simulink model "sampleModel1746"  (R2023a)
settings: Solver=VariableStepAuto  StartTime=0.0  StopTime=10.0  RelTol=1e-3
libraries: hdlsllib x2
settings Model: Creator=user1  LastModifiedBy=user1

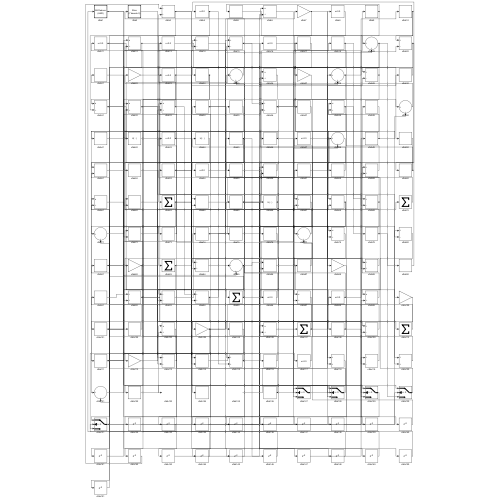
[thumbnail: Simulink's stored preview of the top-level diagram]
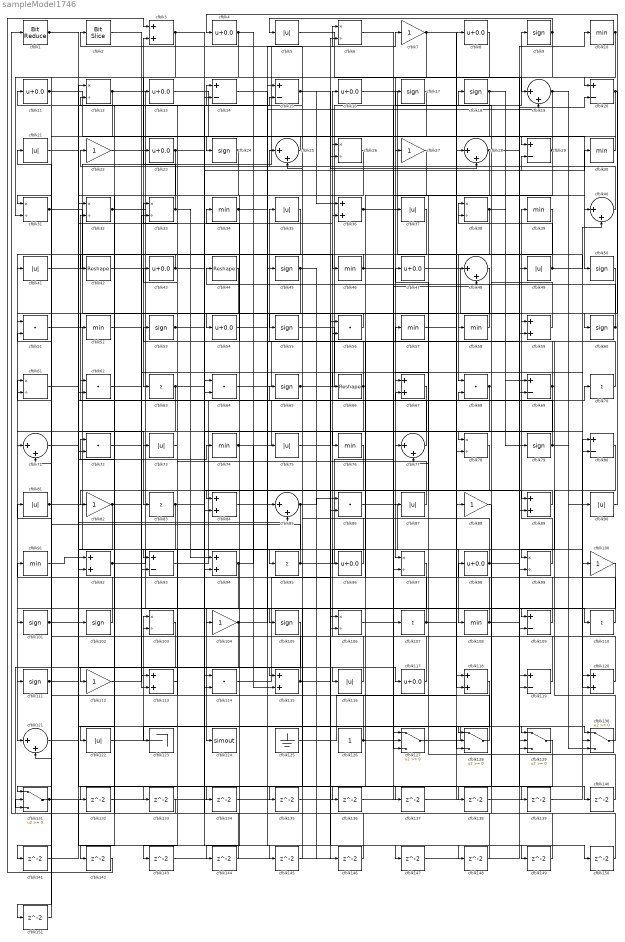
== system sampleModel1746 ==
  cfblk1 : hdlsllib/Logic and Bit Operations/Bit Reduce  mode=AND
  cfblk{10,30,34,39,46,52,57..58,74,76,91,108} (12 alike) : MinMax
  cfblk{7,22,27,82,88,100,104,112} (8 alike) : Gain
  cfblk{9,17..18,24,45,50,53,55,60,65,79,101..102,105,111} (15 alike) : Signum
  cfblk{6,12,26,31..33,38,61,78,97,99,103,106} (13 alike) : Product  Inputs=*/  RndMeth=Zero  SaturateOnIntegerOverflow=on
  cfblk{63,70,83,95,107,110} (6 alike) : Sum  Inputs=+
  cfblk{14..15,20,29,69,80,93,109,119} (9 alike) : Sum  Inputs=+-
  cfblk{4,8,11,13,16,23,43,47,54,96,98,117} (12 alike) : Bias  Bias=0.0  SaturateOnIntegerOverflow=off
  cfblk{3,36,59,67,84,89,92,94,113,115,118,120} (12 alike) : Sum
  cfblk{51,56,62,64,68,72,86,114} (8 alike) : DotProduct  OutDataTypeStr=Inherit: Inherit via internal rule
  cfblk{5,21,35,37,41,49,73,75,81,87,90,116,122} (13 alike) : Abs  SaturateOnIntegerOverflow=off
  cfblk{19,25,28,40,48,71,77,85,121} (9 alike) : Sum  Inputs=|++
  cfblk123 : Terminator
  cfblk124 : ToWorkspace  VariableName=simout  SaveFormat=Timeseries  SampleTime=-1
  cfblk125 : Ground
  cfblk126 : Constant  SampleTime=-1
  cfblk{127..131} (5 alike) : Switch  SaturateOnIntegerOverflow=off  InputSameDT=off
  cfblk{132..151} (20 alike) : Delay  SampleTime=1
  cfblk2 : hdlsllib/Logic and Bit Operations/Bit Slice  lidx=7  ridx=0
  cfblk42 : Reshape
  cfblk44 : Reshape
  cfblk66 : Reshape
  wires:
  cfblk8/1 -> cfblk97/1
  cfblk120/1 -> cfblk47/1
  cfblk24/1 -> cfblk52/1, cfblk132/1
  cfblk9/1 -> cfblk5/1, cfblk31/1
  cfblk69/1 -> cfblk35/1, cfblk86/2
  cfblk74/1 -> cfblk70/1, cfblk7/1
  cfblk99/1 -> cfblk39/1
  cfblk16/1 -> cfblk68/1
  cfblk32/1 -> cfblk109/1, cfblk64/2
  cfblk31/1 -> cfblk54/1, cfblk14/1
  cfblk91/1 -> cfblk92/1
  cfblk25/1 -> cfblk24/1
  cfblk40/1 -> cfblk22/1
  cfblk117/1 -> cfblk16/1
  cfblk104/1 -> cfblk57/1, cfblk110/1, cfblk133/1, cfblk134/1
  cfblk90/1 -> cfblk4/1
  cfblk65/1 -> cfblk9/1, cfblk97/2, cfblk128/3
  cfblk45/1 -> cfblk121/1, cfblk84/2, cfblk146/1
  cfblk125/1 -> cfblk28/1
  cfblk36/1 -> cfblk100/1, cfblk40/1
  cfblk60/1 -> cfblk44/1, cfblk51/1
  cfblk76/1 -> cfblk112/1
  cfblk12/1 -> cfblk66/1, cfblk62/2
  cfblk94/1 -> cfblk121/2, cfblk75/1
  cfblk107/1 -> cfblk8/1, cfblk72/1
  cfblk23/1 -> cfblk78/1, cfblk72/2
  cfblk35/1 -> cfblk111/1
  cfblk92/1 -> cfblk95/1, cfblk118/2
  cfblk4/1 -> cfblk63/1, cfblk115/2
  cfblk13/1 -> cfblk50/1
  cfblk28/1 -> cfblk67/1, cfblk20/2
  cfblk127/1 -> cfblk130/1
  cfblk58/1 -> cfblk26/1
  cfblk46/1 -> cfblk41/1, cfblk69/2
  cfblk39/1 -> cfblk77/1
  cfblk7/1 -> cfblk89/1, cfblk14/2
  cfblk33/1 -> cfblk3/2, cfblk94/1
  cfblk131/1 -> cfblk26/2, cfblk145/1
  cfblk53/1 -> cfblk109/2, cfblk149/1
  cfblk29/1 -> cfblk37/1, cfblk23/1
  cfblk81/1 -> cfblk120/1, cfblk93/1
  cfblk122/1 -> cfblk103/1
  cfblk15/1 -> cfblk28/2, cfblk36/1
  cfblk114/1 -> cfblk56/1
  cfblk59/1 -> cfblk17/1
  cfblk49/1 -> cfblk38/1, cfblk40/2
  cfblk41/1 -> cfblk6/1
  cfblk86/1 -> cfblk108/1
  cfblk38/1 -> cfblk58/1, cfblk69/1
  cfblk128/1 -> cfblk81/1
  cfblk62/1 -> cfblk113/1
  cfblk100/1 -> cfblk124/1
  cfblk17/1 -> cfblk71/1
  cfblk66/1 -> cfblk34/1, cfblk151/1
  cfblk55/1 -> cfblk107/1
  cfblk108/1 -> cfblk56/2, cfblk140/1
  cfblk19/1 -> cfblk29/1, cfblk90/1, cfblk94/2
  cfblk85/1 -> cfblk123/1, cfblk86/1, cfblk93/2
  cfblk105/1 -> cfblk131/1
  cfblk63/1 -> cfblk83/1, cfblk29/2, cfblk129/3
  cfblk68/1 -> cfblk78/2, cfblk96/1
  cfblk109/1 -> cfblk61/1
  cfblk57/1 -> cfblk30/1
  cfblk61/1 -> cfblk102/1
  cfblk30/1 -> cfblk27/1
  cfblk93/1 -> cfblk15/1
  cfblk82/1 -> cfblk92/2, cfblk116/1
  cfblk10/1 -> cfblk20/1, cfblk129/2
  cfblk56/1 -> cfblk55/1
  cfblk116/1 -> cfblk21/1
  cfblk44/1 -> cfblk122/1
  cfblk47/1 -> cfblk119/2
  cfblk77/1 -> cfblk32/2
  cfblk3/1 -> cfblk114/1, cfblk31/2, cfblk139/1
  cfblk51/1 -> cfblk114/2
  cfblk73/1 -> cfblk13/1
  cfblk101/1 -> cfblk67/2, cfblk129/1, cfblk36/2
  cfblk130/1 -> cfblk59/1
  cfblk14/1 -> cfblk85/1
  cfblk21/1 -> cfblk73/1
  cfblk121/1 -> cfblk85/2
  cfblk42/1 -> cfblk120/2
  cfblk72/1 -> cfblk68/2
  cfblk119/1 -> cfblk25/1
  cfblk113/1 -> cfblk53/1
  cfblk64/1 -> cfblk49/1
  cfblk27/1 -> cfblk76/1
  cfblk80/1 -> cfblk99/1
  cfblk115/1 -> cfblk62/1, cfblk150/1
  cfblk110/1 -> cfblk98/1
  cfblk83/1 -> cfblk113/2, cfblk15/2
  cfblk50/1 -> cfblk87/1
  cfblk22/1 -> cfblk118/1
  cfblk70/1 -> cfblk43/1
  cfblk20/1 -> cfblk101/1, cfblk60/1
  cfblk102/1 -> cfblk91/1
  cfblk52/1 -> cfblk104/1
  cfblk89/1 -> cfblk84/1
  cfblk98/1 -> cfblk2/1, cfblk10/1
  cfblk87/1 -> cfblk33/1
  cfblk6/1 -> cfblk127/2
  cfblk96/1 -> cfblk11/1
  cfblk71/1 -> cfblk12/1
  cfblk126/1 -> cfblk103/2, cfblk18/1
  cfblk111/1 -> cfblk128/1, cfblk74/1, cfblk115/1
  cfblk43/1 -> cfblk89/2, cfblk42/1
  cfblk95/1 -> cfblk48/2, cfblk51/2
  cfblk37/1 -> cfblk82/1
  cfblk112/1 -> cfblk33/2
  cfblk48/1 -> cfblk106/2
  cfblk2/1 -> cfblk105/1
  cfblk103/1 -> cfblk131/3
  cfblk5/1 -> cfblk19/1
  cfblk106/1 -> cfblk128/2
  cfblk18/1 -> cfblk127/3, cfblk79/1
  cfblk34/1 -> cfblk80/2, cfblk19/2
  cfblk54/1 -> cfblk45/1
  cfblk11/1 -> cfblk88/1, cfblk137/1
  cfblk79/1 -> cfblk65/1, cfblk130/3
  cfblk1/1 -> cfblk46/1, cfblk117/1
  cfblk132/1 -> cfblk127/1
  cfblk133/1 -> cfblk1/1
  cfblk134/1 -> cfblk6/2
  cfblk97/1 -> cfblk135/1
  cfblk135/1 -> cfblk48/1
  cfblk78/1 -> cfblk136/1
  cfblk136/1 -> cfblk119/1
  cfblk137/1 -> cfblk59/2
  cfblk88/1 -> cfblk138/1
  cfblk138/1 -> cfblk80/1
  cfblk139/1 -> cfblk130/2
  cfblk140/1 -> cfblk77/2
  cfblk67/1 -> cfblk141/1
  cfblk141/1 -> cfblk32/1
  cfblk129/1 -> cfblk142/1
  cfblk142/1 -> cfblk3/1
  cfblk118/1 -> cfblk143/1
  cfblk143/1 -> cfblk106/1
  cfblk26/1 -> cfblk144/1
  cfblk144/1 -> cfblk131/2
  cfblk145/1 -> cfblk25/2
  cfblk146/1 -> cfblk12/2
  cfblk84/1 -> cfblk147/1
  cfblk147/1 -> cfblk99/2
  cfblk75/1 -> cfblk148/1
  cfblk148/1 -> cfblk61/2
  cfblk149/1 -> cfblk64/1
  cfblk150/1 -> cfblk38/2
  cfblk151/1 -> cfblk71/2
